simulink model "ball_beam_retroazionato_simulink"  (R2020a)
settings: Solver=VariableStepAuto  StartTime=0.0  StopTime=10.0  FixedStep=0.01  MaxStep=0.01  RelTol=1e-3
values from neighbouring files (symbols this model uses):
  amp = amp-0.1    (= 0.1)    [prova_regolatore.m]
  den_R = cell2mat(R.Denominator)    [prova_regolatore.m]
  k = (DATI.m*DATI.g*DATI.d) / (m_eq * DATI.L)    [prova_regolatore.m]
  num_R = cell2mat(R.Numerator)    [prova_regolatore.m]
  r_fin = str2double(r_fin_cell{1, 1})    [prova_regolatore.m]
  wd = str2double(wd_cell{1, 1})    [prova_regolatore.m]
settings Model: Creator=peter  LastModifiedBy=peter
settings DataIOCC: SaveFormat=Array  SignalLogging=off  DSMLogging=off  ReturnWorkspaceOutputs=off

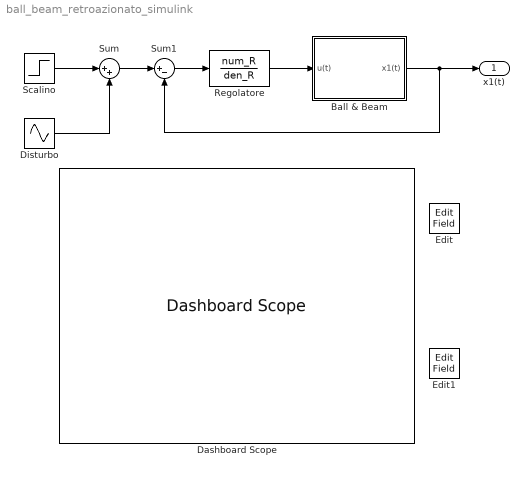
== system ball_beam_retroazionato_simulink ==
  Ball & Beam : Subsystem  VariantControl=Choice
  Dashboard Scope : DashboardScope
  Disturbo : Sin  Amplitude=amp  Frequency=wd  SampleTime=0
  Edit : EditField  LabelPosition=Bottom  ShowInitialText=on  Alignment=Center
  Edit1 : EditField  LabelPosition=Bottom  ShowInitialText=on  Alignment=Center
  Regolatore : TransferFcn  Numerator=num_R  Denominator=den_R
  Scalino : Step  Time=0  After=r_fin  SampleTime=0.01
  Sum : Sum  Inputs=|++
  Sum1 : Sum  Inputs=|+-
  x1(t) : Outport
  wires:
  Regolatore/1 -> Ball & Beam/1(u(t))
  Ball & Beam/1(x1(t)) -> Sum1/2, x1(t)/1
  Sum/1 -> Sum1/1
  Sum1/1 -> Regolatore/1
  Scalino/1 -> Sum/1
  Disturbo/1 -> Sum/2

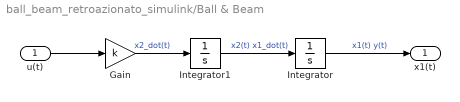
== system ball_beam_retroazionato_simulink/Ball & Beam ==
  u(t) : Inport
  Gain : Gain  Gain=k
  Integrator : Integrator
  Integrator1 : Integrator
  x1(t) : Outport
  wires:
  Integrator/1 -> x1(t)/1  "x1(t) y(t)"
  u(t)/1 -> Gain/1
  Integrator1/1 -> Integrator/1  "x2(t) x1_dot(t)"
  Gain/1 -> Integrator1/1  "x2_dot(t)"
